simulink model "Simulink_model"  (R2024b)
settings: Solver=VariableStepAuto  StartTime=0.0  StopTime=20  FixedStep=Ts  RelTol=1e-3
values from neighbouring files (symbols this model uses):
  A = [0, 1; -2, -40]    [Script.m]
  B = [0; 40]    [Script.m]
  C = [1, 0]    [Script.m]
  D = 0    [Script.m]
  Gamma_obs = [Gamma, L]    [Script.m]
  H_obs = eye(n)    [Script.m]
  J_obs = zeros(n, m+p)    [Script.m]
  K = Ke(2:n+1)    [Script.m]
  Ki = Ke(1)    [Script.m]
  Nu = N(n+1:end)    [Script.m]
  Nx = N(1:n)    [Script.m]
  Phi_obs = Phi-L*H    [Script.m]
  Ts = 0.01e-3    (= 1e-05)    [Script.m]
undefined symbols (not defined in the file or in its folder): DiscIntNeverNeededParam
settings Model: Creator=andre  LastModifiedBy=Enrico 2

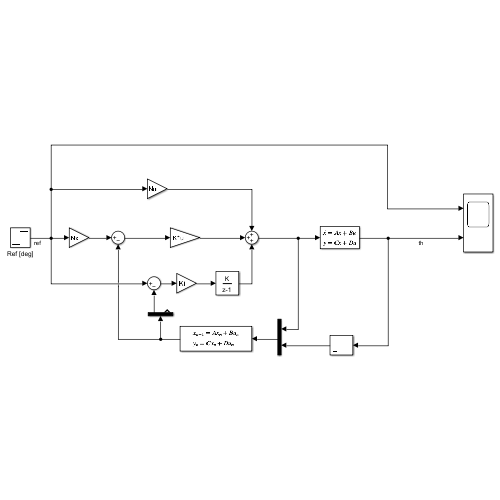
[thumbnail: Simulink's stored preview of the top-level diagram]
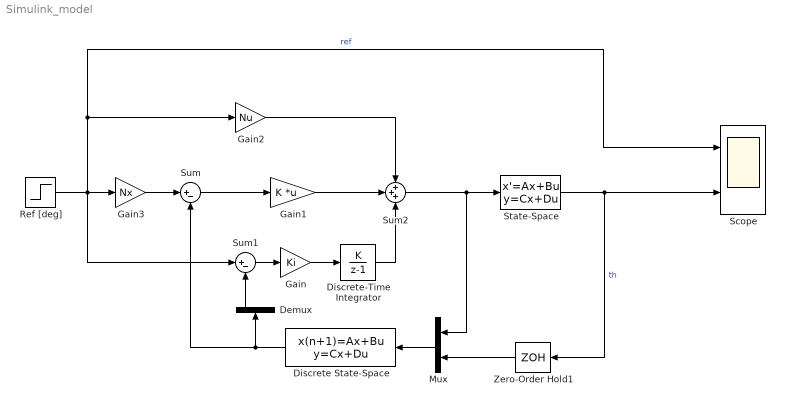
== system Simulink_model ==
  Demux : Demux  Outputs=2
  Discrete State-Space : DiscreteStateSpace  A=Phi_obs  B=Gamma_obs  C=H_obs  D=J_obs  SampleTime=Ts
  Discrete-Time Integrator : DiscreteIntegrator  IntegratorMethod=Accumulation: Forward Euler  SampleTime=Ts  ICPrevOutput=DiscIntNeverNeededParam  ICPrevScaledInput=DiscIntNeverNeededParam
  Gain : Gain  Gain=Ki
  Gain1 : Gain  Gain=K  Multiplication=Matrix(K*u)
  Gain2 : Gain  Gain=Nu
  Gain3 : Gain  Gain=Nx
  Mux : Mux  Inputs=2
  Ref [deg] : Step  After=100  SampleTime=0
  Scope : Scope  NumInputPorts=2
  State-Space : StateSpace  A=A  B=B  C=C  D=D  InitialCondition=0
  Sum : Sum  Inputs=|+-
  Sum1 : Sum  Inputs=|+-
  Sum2 : Sum  Inputs=+++
  Zero-Order Hold1 : ZeroOrderHold  SampleTime=Ts
  wires:
  State-Space/1 -> Scope/2, Zero-Order Hold1/1  "th"
  Mux/1 -> Discrete State-Space/1
  Zero-Order Hold1/1 -> Mux/2
  Gain1/1 -> Sum2/2
  Gain2/1 -> Sum2/1
  Gain3/1 -> Sum/1
  Sum2/1 -> Mux/1, State-Space/1
  Ref [deg]/1 -> Gain3/1, Scope/1, Gain2/1, Sum1/1  "ref"
  Discrete State-Space/1 -> Demux/1, Sum/2
  Demux/1 -> Sum1/2
  Discrete-Time Integrator/1 -> Sum2/3
  Sum1/1 -> Gain/1
  Gain/1 -> Discrete-Time Integrator/1
  Sum/1 -> Gain1/1
